simulink model "IM_D04_VFD_5HP"  (R2024a)
settings: Solver=VariableStepAuto  StartTime=0.0  StopTime=10  RelTol=1e-3
libraries: spsMosfetLib x6, simulink x2, spsAsynchronousMachineSIUnitsLib x1, spsDCVoltageSourceLib x1, spsGroundLib x1, spsThreePhaseVIMeasurementLib x1, sps_lib x1
settings Model: Creator=pc  LastModifiedBy=pc

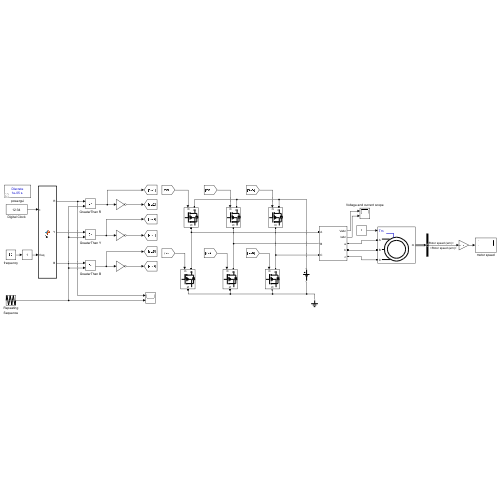
[thumbnail: Simulink's stored preview of the top-level diagram]
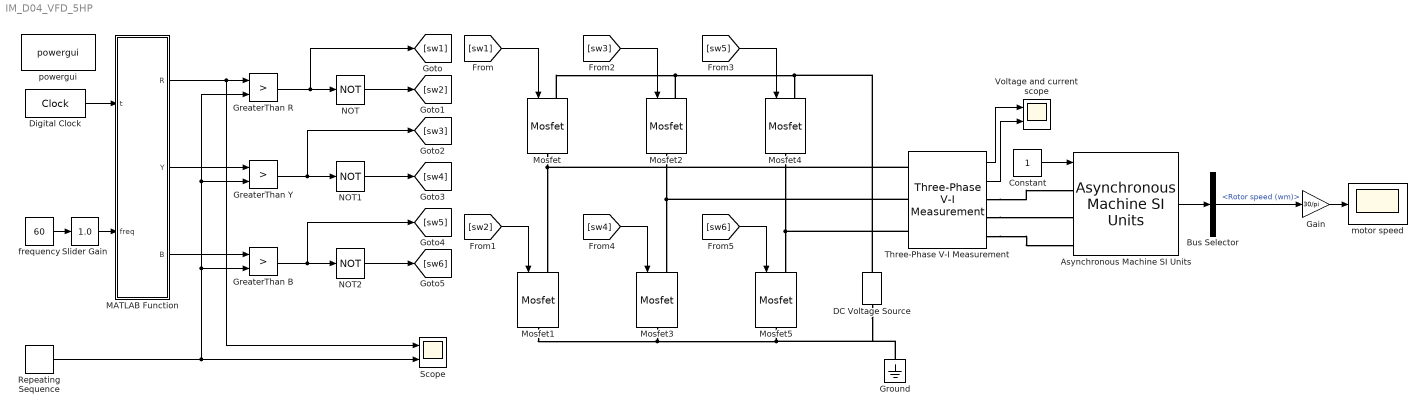
== system IM_D04_VFD_5HP ==
  Asynchronous Machine SI Units : spsAsynchronousMachineSIUnitsLib/Asynchronous Machine SI Units  RotorType=Squirrel-cage  PresetModel="14:  200 HP 575 V 60Hz 1785 RPM"  MechanicalLoad=Torque Tm  ShowDetailedParameters=on  ReferenceFrame=Rotor  Units=SI  MeasurementBus=off  NominalParameters=[1.492e+05 575 60]  VoltageRatio=1  Stator=[0.02475 0.000284]  Rotor=[0.01329 0.000284]  Cage1=[0.4155 0.002066]  Cage2=[0.4168 0.0003495]  Lm=0.01425  Mechanical=[2.6 0.06346 2]  PolePairs=2  InitialConditions=[0 0 0 0 0 0 0 0]  SimulateSaturation=off  Saturation=[14.03593122, 27.81365428, 53.79336849, 72.68890987, 97.98006896, 148.6815601, 215.7428561, 302.9841135, 428.7778367 ; 230, 322, 414, 460, 506, 552, 598, 644, 690]  LoadFlowParameters=1492000  TsPowergui=0  TsBlock=-1  IterativeModel=Trapezoidal non iterative  IterativeDiscreteModel=Trapezoidal non iterative  Pmec=746
  Bus Selector : BusSelector  OutputSignals=Mechanical.Rotor speed (wm)
  Constant : Constant
  DC Voltage Source : spsDCVoltageSourceLib/DC Voltage Source  Amplitude=575  Measurements=None
  Digital Clock : DigitalClock  SampleTime=1e-05
  Gain : Gain  Gain=30/pi
  GreaterThan B : RelationalOperator  Operator=>  OutDataTypeStr=boolean  RndMeth=Simplest  InputSameDT=off
  GreaterThan R : RelationalOperator  Operator=>  OutDataTypeStr=boolean  RndMeth=Simplest  InputSameDT=off
  GreaterThan Y : RelationalOperator  Operator=>  OutDataTypeStr=boolean  RndMeth=Simplest  InputSameDT=off
  Ground : spsGroundLib/Ground  LConnTagsString=a
  MATLAB Function : MATLAB Function  TreatAsAtomicUnit=on
  Mosfet{,1..5} (6 alike) : spsMosfetLib/Mosfet  Ron=0.1  Lon=0  Rd=0.01  Vfd=0  IC=0  Rs=1e5  Cs=inf  Measurements=off
  NOT : Logic  Operator=NOT  IconShape=distinctive  AllPortsSameDT=off  OutDataTypeStr=boolean
  NOT1 : Logic  Operator=NOT  IconShape=distinctive  AllPortsSameDT=off  OutDataTypeStr=boolean
  NOT2 : Logic  Operator=NOT  IconShape=distinctive  AllPortsSameDT=off  OutDataTypeStr=boolean
  Repeating Sequence : simulink/Sources/Repeating Sequence  rep_seq_t=[0 0.25 0.5 0.75 1]* (1/5000)  rep_seq_y=[0 1 0 -1 0]
  Scope : Scope  NumInputPorts=2
  Slider Gain : simulink/Math Operations/Slider Gain  gain=1.0  low=0  high=1
  Three-Phase V-I Measurement : spsThreePhaseVIMeasurementLib/Three-Phase V-I Measurement  VoltageMeasurement=phase-to-ground  SetLabelV=off  LabelV=Vabc  Vpu=off  VpuLL=off  CurrentMeasurement=yes  SetLabelI=off  LabelI=Iabc  Ipu=off  Pbase=100e6  Vbase=500e3  OutputType=Complex  PhasorSimulation=off  PSBequivalent=0
  Voltage and current scope : Scope  NumInputPorts=2
  frequency : Constant  Value=60
  motor speed : Scope
  powergui : sps_lib/powergui  Priority=1  SimulationMode=Discrete  SampleTime=1e-05  frequency=60  Iterations=50  frequencyindice=60  Pbase=100e6  ErrMax=1e-4  UnitsV=kV  UnitsW=MW  buscounter=0  FunctionMessages=off  echomessages=off  EnableUseOfTLC=off  CurrentSourceSwitches=off  DisableSnubberDevices=off  DisableRonSwitches=off  DisableVfSwitches=off  DisplayEquations=off  AutomaticDiscreteSolvers=off  SolverType=Tustin/Backward Euler (TBE)  Interpol=off  ExternalGateDelay=off  methode=off  Ts=100  x0status=blocks  SPID=on  SwTol=0  HookPort=off  NonlinearTolerance=1e-4  nMaxIteration=100  ContinueOnMaxIteration=off  RestoreLinks=warning  ResistiveCurrentMeasurement=off  Frange=[0:2:500]  Ylog=off  Xlog=on  ShowGrid=off  save=off  variable=ZData  structure=0  ZoomFFT=off  StartTime=0.0  cycles=1  DisplayStyle=1  fundamental=60  FreqAxis=off  MaxFrequency=1000  frequencyindicesteady=1  RmsSteady=1  display=off
  wires:
  MATLAB Function/1(R) -> Scope/1, GreaterThan R/1
  GreaterThan R/1 -> [sw1], NOT/1
  frequency/1 -> Slider Gain/1
  Slider Gain/1 -> MATLAB Function/2(freq)
  GreaterThan Y/1 -> [sw3], NOT1/1
  Repeating Sequence/1 -> Scope/2, GreaterThan R/2, GreaterThan Y/2, GreaterThan B/2
  MATLAB Function/2(Y) -> GreaterThan Y/1
  MATLAB Function/3(B) -> GreaterThan B/1
  Digital Clock/1 -> MATLAB Function/1(t)
  NOT/1 -> [sw2]
  NOT2/1 -> [sw6]
  GreaterThan B/1 -> [sw5], NOT2/1
  NOT1/1 -> [sw4]
  [sw1] -> Mosfet/1
  [sw2] -> Mosfet1/1
  [sw3] -> Mosfet2/1
  [sw5] -> Mosfet4/1
  [sw4] -> Mosfet3/1
  [sw6] -> Mosfet5/1
  Constant/1 -> Asynchronous Machine SI Units/1
  Bus Selector/1 -> Gain/1  "<Rotor speed (wm)>"
  Three-Phase V-I Measurement/2 -> Voltage and current scope/2
  Asynchronous Machine SI Units/1 -> Bus Selector/1
  Gain/1 -> motor speed/1
  Three-Phase V-I Measurement/1 -> Voltage and current scope/1
  connections:
  Mosfet/LConn1 -- Mosfet2/LConn1 -- DC Voltage Source/RConn1 -- Mosfet4/LConn1
  Mosfet2/RConn1 -- Three-Phase V-I Measurement/LConn2 -- Mosfet3/LConn1
  Mosfet4/RConn1 -- Three-Phase V-I Measurement/LConn3 -- Mosfet5/LConn1
  Mosfet/RConn1 -- Three-Phase V-I Measurement/LConn1 -- Mosfet1/LConn1
  Mosfet1/RConn1 -- Mosfet3/RConn1 -- Ground/LConn1 -- DC Voltage Source/LConn1 -- Mosfet5/RConn1
  Three-Phase V-I Measurement/RConn2 -- Asynchronous Machine SI Units/LConn2
  Three-Phase V-I Measurement/RConn1 -- Asynchronous Machine SI Units/LConn1
  Three-Phase V-I Measurement/RConn3 -- Asynchronous Machine SI Units/LConn3

== matlab function IM_D04_VFD_5HP/MATLAB Function ==
  data: t input; R output; freq input; Y output; B output
function [R,Y,B] = fcn(t, freq)
omega = 2*pi*freq;
R = sin(omega*t)*freq/60;
B = sin(omega*t + 120*pi/180)*freq/60;
Y = sin(omega*t + 240*pi/180)*freq/60;
